simulink model "Motor"  (R2024a)
settings: Solver=VariableStepAuto  StartTime=0.0  StopTime=10.0  RelTol=1e-3
model workspace (MATLAB code in the model file):
  | MotorParams;
  | WheelParams;
undefined symbols (not defined in the file): motor_gyration, motor_resistance, wheel_inertia
settings Model: Creator=Marij  LastModifiedBy=Marij
settings OptimizationCC: UseDivisionForNetSlopeComputation=on
settings ModelReferenceCC: ModelReferenceMinAlgLoopOccurrences=on

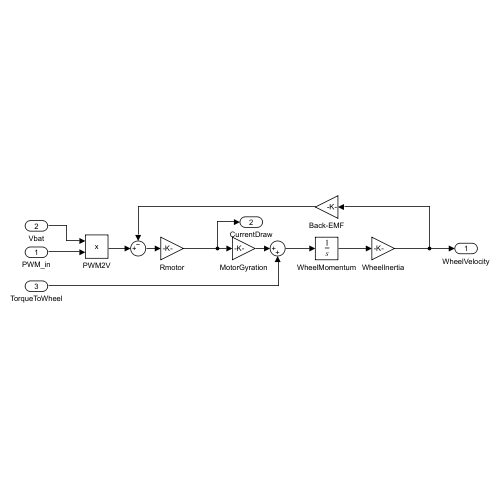
[thumbnail: Simulink's stored preview of the top-level diagram]
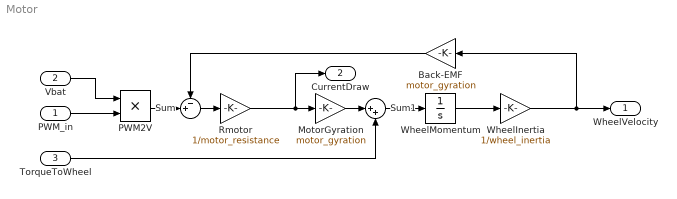
== system Motor ==
  PWM_in : Inport
  Vbat : Inport  Port=2
  TorqueToWheel : Inport  Port=3
  Back-EMF : Gain  Gain=motor_gyration
  MotorGyration : Gain  Gain=motor_gyration
  PWM2V : Product
  Rmotor : Gain  Gain=1/motor_resistance
  Sum : Sum  Inputs=-+|
  Sum1 : Sum  Inputs=|++
  WheelInertia : Gain  Gain=1/wheel_inertia
  WheelMomentum : Integrator
  WheelVelocity : Outport  Unit=rad/s
  CurrentDraw : Outport  Port=2  Unit=A  PortDimensions=1
  wires:
  PWM_in/1 -> PWM2V/2
  Vbat/1 -> PWM2V/1
  WheelMomentum/1 -> WheelInertia/1
  Back-EMF/1 -> Sum/1
  PWM2V/1 -> Sum/2
  WheelInertia/1 -> WheelVelocity/1, Back-EMF/1
  Sum/1 -> Rmotor/1
  Rmotor/1 -> CurrentDraw/1, MotorGyration/1
  Sum1/1 -> WheelMomentum/1
  TorqueToWheel/1 -> Sum1/2
  MotorGyration/1 -> Sum1/1
